simulink model "AtoD_test_FBand"  (R2016b)
settings: Solver=ode45  StartTime=0.0  StopTime=10.0  RelTol=1e-3
values from neighbouring files (symbols this model uses):
  Ts = 1/Fadc    (= 3.25520833333e-09)    [setupCryoFPGA.m]    (also in setupCryoFPGA_CMB.m; setupCryoFPGAorig.m = 3.2e-09)
undefined symbols (not defined in the file or in its folder): AXI4, Lite
libraries: xbsIndex_r4 x78
settings Model: Creator=ssmith  LastModifiedBy=jedu
settings DataIOCC: LimitDataPoints=on  SaveFormat=Array
settings OptimizationCC: BlockReduction=off  BooleanDataType=off  LifeSpan=inf
settings DebuggingCC: SaveWithParameterizedLinksMsg=none  UnderspecifiedInitializationDetection=Classic  MergeDetectMultiDrivingBlocksExec=none  SignalResolutionControl=TryResolveAllWithWarning  SFUnexpectedBacktrackingDiag=warning  SFNoUnconditionalDefaultTransitionDiag=warning  SFExecutionAtInitializationDiag=none
settings HardwareCC: ProdBitPerPointer=32  ProdBitPerSizeT=32  ProdBitPerPtrDiffT=32  ProdLargestAtomicFloat=None  ProdIntDivRoundTo=Undefined  ProdEndianess=Unspecified  ProdWordSize=32  ProdHWDeviceType=32-bit Generic  TargetUnknown=on
settings ModelReferenceCC: PropagateSignalLabelsOutOfModel=off
settings GRTTargetCC: TargetLangStandard=C89/C90 (ANSI)  GeneratePreprocessorConditionals=Disable all
settings ConfigComp: CovMetricSettings=dw  CovHtmlReporting=on  CovSaveCumulativeToWorkspaceVar=on  CovSaveSingleToWorkspaceVar=on  CovExternalEMLEnable=off  CovSFcnEnable=off

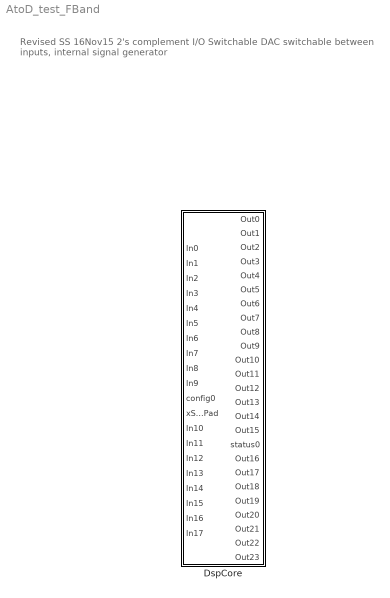
== system AtoD_test_FBand ==
  note: Revised SS 16Nov15
      | 	2's complement I/O
      | 	Switchable DAC switchable between inputs, internal signal generator
  DspCore : Subsystem

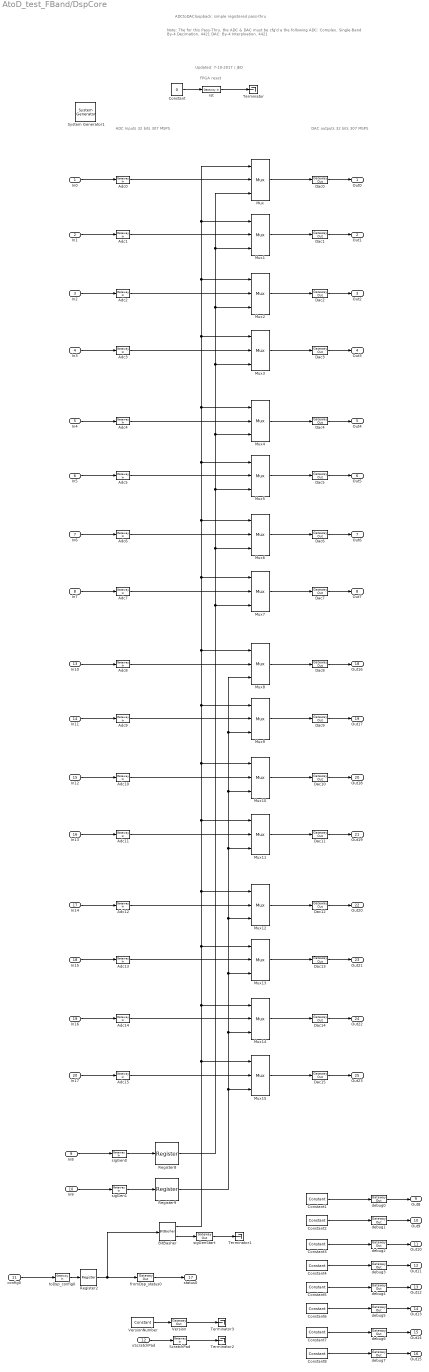
== system AtoD_test_FBand/DspCore ==
  note: Updated: 7-10-2017 / JED
  note: ADCtoDACloopback: simple registered pass-thru
  note: DAC outputs
      | 32 bits
      | 307 MSPS
  note: ADC Inputs
      | 32 bits
      | 307 MSPS
  note: FPGA reset
  note: Note: The for this Pass-Thru, the ADC & DAC must be cfg'd a the following
      |
      | ADC: Complex, Single-Band By-4 Decimation, 4421
      | DAC: By-4 Interploation, 4421
  In0 : Inport
  In1 : Inport  Port=2
  In2 : Inport  Port=3
  In3 : Inport  Port=4
  In4 : Inport  Port=5
  In5 : Inport  Port=6
  In6 : Inport  Port=7
  In7 : Inport  Port=8
  In8 : Inport  Port=9
  In9 : Inport  Port=10
  config0 : Inport  Port=11
  xScratchPad : Inport  Port=12
  In10 : Inport  Port=13
  In11 : Inport  Port=14
  In12 : Inport  Port=15
  In13 : Inport  Port=16
  In14 : Inport  Port=17
  In15 : Inport  Port=18
  In16 : Inport  Port=19
  In17 : Inport  Port=20
  " System Generator1" : xbsIndex_r4/ System Generator  Tag=genX  xilinxfamily=kintexu  part=xcku060  speed=-2-e  package=ffva1156  synthesis_tool=Vivado  clock_wrapper=Clock Enables  directory=./netlist  proj_type=Vivado  Synth_file=Vivado Synthesis Defaults  Impl_file=Vivado Implementation Defaults  testbench=off  simulink_period=Ts  sysclk_period=Ts*1e9  dcm_input_clock_period=10  incr_netlist=off  trim_vbits=Everywhere in SubSystem  dbl_ovrd=According to Block Masks  core_generation=According to Block Masks  run_coregen=off  deprecated_control=off  eval_field=0  block_type=sysgen
  Adc{0..15} (16 alike) : xbsIndex_r4/Gateway In  gui_display_data_type=Fixed-point  arith_type=Unsigned  n_bits=32  bin_pt=0  preci_type=Single  exp_width=8  frac_width=24  rows=1  columns=1  quantization=Truncate  overflow=Wrap  period=Ts  UseAsADC=off  ADCChannel='1'  interface=None  automatic_assignment=on  address_offset=hex2dec('00')  intf_name=''  intf_description=''  default_value=0  timing_constraint=None  locs_specified=off  LOCs={}  io_standard={}  inherit_from_input=off  hdl_port=on  dbl_ovrd=off  block_type=gatewayin
  BitBasher : xbsIndex_r4/BitBasher  bitexpr=|  display_expr=off  sr_1=sel  arith_type1=Unsigned  bin_pt1=0  sr_2=start  arith_type2=Unsigned  bin_pt2=0  sr_3=3  arith_type3=Unsigned  bin_pt3=0  sr_4=4  arith_type4=Unsigned  bin_pt4=0  dbl_ovrd=off  block_type=bitbasher
      | sel={a[0]}
      | start={a[1]}
  Constant : Constant  Value=0
  Constant1 : xbsIndex_r4/Constant  const=0  gui_display_data_type=Fixed-point  arith_type=Unsigned  n_bits=32  bin_pt=0  preci_type=Single  exp_width=8  frac_width=24  explicit_period=off  period=1  equ=P=C  opselect=C  inp2=PCIN>>17  opr=+  inp1=P  carry=CIN  dbl_ovrd=off  block_type=constant
  Constant2 : xbsIndex_r4/Constant  const=1  gui_display_data_type=Fixed-point  arith_type=Unsigned  n_bits=32  bin_pt=0  preci_type=Single  exp_width=8  frac_width=24  explicit_period=off  period=1  equ=P=C  opselect=C  inp2=PCIN>>17  opr=+  inp1=P  carry=CIN  dbl_ovrd=off  block_type=constant
  Constant3 : xbsIndex_r4/Constant  const=2  gui_display_data_type=Fixed-point  arith_type=Unsigned  n_bits=32  bin_pt=0  preci_type=Single  exp_width=8  frac_width=24  explicit_period=off  period=1  equ=P=C  opselect=C  inp2=PCIN>>17  opr=+  inp1=P  carry=CIN  dbl_ovrd=off  block_type=constant
  Constant4 : xbsIndex_r4/Constant  const=3  gui_display_data_type=Fixed-point  arith_type=Unsigned  n_bits=32  bin_pt=0  preci_type=Single  exp_width=8  frac_width=24  explicit_period=off  period=1  equ=P=C  opselect=C  inp2=PCIN>>17  opr=+  inp1=P  carry=CIN  dbl_ovrd=off  block_type=constant
  Constant5 : xbsIndex_r4/Constant  const=4  gui_display_data_type=Fixed-point  arith_type=Unsigned  n_bits=32  bin_pt=0  preci_type=Single  exp_width=8  frac_width=24  explicit_period=off  period=1  equ=P=C  opselect=C  inp2=PCIN>>17  opr=+  inp1=P  carry=CIN  dbl_ovrd=off  block_type=constant
  Constant6 : xbsIndex_r4/Constant  const=5  gui_display_data_type=Fixed-point  arith_type=Unsigned  n_bits=32  bin_pt=0  preci_type=Single  exp_width=8  frac_width=24  explicit_period=off  period=1  equ=P=C  opselect=C  inp2=PCIN>>17  opr=+  inp1=P  carry=CIN  dbl_ovrd=off  block_type=constant
  Constant7 : xbsIndex_r4/Constant  const=6  gui_display_data_type=Fixed-point  arith_type=Unsigned  n_bits=32  bin_pt=0  preci_type=Single  exp_width=8  frac_width=24  explicit_period=off  period=1  equ=P=C  opselect=C  inp2=PCIN>>17  opr=+  inp1=P  carry=CIN  dbl_ovrd=off  block_type=constant
  Constant8 : xbsIndex_r4/Constant  const=7  gui_display_data_type=Fixed-point  arith_type=Unsigned  n_bits=32  bin_pt=0  preci_type=Single  exp_width=8  frac_width=24  explicit_period=off  period=1  equ=P=C  opselect=C  inp2=PCIN>>17  opr=+  inp1=P  carry=CIN  dbl_ovrd=off  block_type=constant
  Dac{0..15} (16 alike) : xbsIndex_r4/Gateway Out  inherit_from_input=on  hdl_port=on  rows=1  columns=1  UseAsDAC=off  DACChannel='1'  interface=None  automatic_assignment=on  address_offset=hex2dec('00')  intf_name=''  intf_description=''  timing_constraint=None  locs_specified=off  LOCs={}  io_standard={}  block_type=gatewayout
  Mux{,1..15} (16 alike) : xbsIndex_r4/Mux  inputs=2  en=off  latency=1  precision=Full  arith_type=Unsigned  n_bits=16  bin_pt=14  quantization=Truncate  overflow=Wrap  dbl_ovrd=off  block_type=mux
  Register2 : xbsIndex_r4/Register  init=0  rst=off  en=off  dbl_ovrd=off  block_type=register
  Register8 : xbsIndex_r4/Register  init=0  rst=off  en=off  dbl_ovrd=off  block_type=register
  Register9 : xbsIndex_r4/Register  init=0  rst=off  en=off  dbl_ovrd=off  block_type=register
  ScratchPad : xbsIndex_r4/Gateway In  gui_display_data_type=Fixed-point  arith_type=Unsigned  n_bits=32  bin_pt=0  preci_type=Single  exp_width=8  frac_width=24  rows=1  columns=1  quantization="Round  (unbiased: +/- Inf)"  overflow=Saturate  period=Ts  UseAsADC=off  ADCChannel='1'  interface=AXI4-Lite  automatic_assignment=off  address_offset=hex2dec('FFC')  intf_name=''  intf_description=''  default_value=0  timing_constraint=None  locs_specified=off  LOCs={}  io_standard={}  inherit_from_input=off  hdl_port=on  dbl_ovrd=off  block_type=gatewayin
  Terminator{,1..3} (4 alike) : Terminator
  Version : xbsIndex_r4/Gateway Out  inherit_from_input=on  hdl_port=on  rows=1  columns=1  UseAsDAC=off  DACChannel='1'  interface=AXI4-Lite  automatic_assignment=off  address_offset=hex2dec('000')  intf_name=''  intf_description=''  timing_constraint=None  locs_specified=off  LOCs={}  io_standard={}  block_type=gatewayout
  VersionNumber : xbsIndex_r4/Constant  const=hex2dec('00000001')  gui_display_data_type=Fixed-point  arith_type=Unsigned  n_bits=32  bin_pt=0  preci_type=Single  exp_width=8  frac_width=24  explicit_period=off  period=1  equ=P=C  opselect=C  inp2=PCIN>>17  opr=+  inp1=P  carry=CIN  dbl_ovrd=off  block_type=constant
  debug{0..7} (8 alike) : xbsIndex_r4/Gateway Out  inherit_from_input=on  hdl_port=on  rows=1  columns=1  UseAsDAC=off  DACChannel='1'  interface=None  automatic_assignment=on  address_offset=hex2dec('00')  intf_name=''  intf_description=''  timing_constraint=None  locs_specified=off  LOCs={}  io_standard={}  block_type=gatewayout
  fromDsp_status0 : xbsIndex_r4/Gateway Out  inherit_from_input=on  hdl_port=on  rows=1  columns=1  UseAsDAC=off  DACChannel='1'  interface=AXI4-Lite  automatic_assignment=off  address_offset=hex2dec('004')  intf_name=''  intf_description=''  timing_constraint=None  locs_specified=off  LOCs={}  io_standard={}  block_type=gatewayout
  rst : xbsIndex_r4/Gateway In  gui_display_data_type=Boolean  arith_type=Boolean  n_bits=16  bin_pt=14  preci_type=Single  exp_width=8  frac_width=24  rows=1  columns=1  quantization="Round  (unbiased: +/- Inf)"  overflow=Saturate  period=Ts  UseAsADC=off  ADCChannel='1'  interface=None  automatic_assignment=on  address_offset=hex2dec('00')  intf_name=''  intf_description=''  default_value=0  timing_constraint=None  locs_specified=off  LOCs={}  io_standard={}  inherit_from_input=off  hdl_port=on  dbl_ovrd=off  block_type=gatewayin
  sigGen0 : xbsIndex_r4/Gateway In  gui_display_data_type=Fixed-point  arith_type=Unsigned  n_bits=32  bin_pt=0  preci_type=Single  exp_width=8  frac_width=24  rows=1  columns=1  quantization=Truncate  overflow=Wrap  period=Ts  UseAsADC=off  ADCChannel='1'  interface=None  automatic_assignment=on  address_offset=hex2dec('00')  intf_name=''  intf_description=''  default_value=0  timing_constraint=None  locs_specified=off  LOCs={}  io_standard={}  inherit_from_input=off  hdl_port=on  dbl_ovrd=off  block_type=gatewayin
  sigGen1 : xbsIndex_r4/Gateway In  gui_display_data_type=Fixed-point  arith_type=Unsigned  n_bits=32  bin_pt=0  preci_type=Single  exp_width=8  frac_width=24  rows=1  columns=1  quantization=Truncate  overflow=Wrap  period=Ts  UseAsADC=off  ADCChannel='1'  interface=None  automatic_assignment=on  address_offset=hex2dec('00')  intf_name=''  intf_description=''  default_value=0  timing_constraint=None  locs_specified=off  LOCs={}  io_standard={}  inherit_from_input=off  hdl_port=on  dbl_ovrd=off  block_type=gatewayin
  sigGenStart : xbsIndex_r4/Gateway Out  inherit_from_input=on  hdl_port=on  rows=1  columns=1  UseAsDAC=off  DACChannel='1'  interface=None  automatic_assignment=off  address_offset=hex2dec('004')  intf_name=''  intf_description=''  timing_constraint=None  locs_specified=off  LOCs={}  io_standard={}  block_type=gatewayout
  toDsp_config0 : xbsIndex_r4/Gateway In  gui_display_data_type=Fixed-point  arith_type=Unsigned  n_bits=32  bin_pt=0  preci_type=Single  exp_width=8  frac_width=24  rows=1  columns=1  quantization="Round  (unbiased: +/- Inf)"  overflow=Saturate  period=Ts  UseAsADC=off  ADCChannel='1'  interface=AXI4-Lite  automatic_assignment=off  address_offset=hex2dec('080')  intf_name=''  intf_description=''  default_value=0  timing_constraint=None  locs_specified=off  LOCs={}  io_standard={}  inherit_from_input=off  hdl_port=on  dbl_ovrd=off  block_type=gatewayin
  Out0 : Outport  OutDataTypeStr=uint32
  Out1 : Outport  Port=2
  Out2 : Outport  Port=3
  Out3 : Outport  Port=4
  Out4 : Outport  Port=5
  Out5 : Outport  Port=6
  Out6 : Outport  Port=7
  Out7 : Outport  Port=8
  Out8 : Outport  Port=9  OutDataTypeStr=uint32
  Out9 : Outport  Port=10  OutDataTypeStr=uint32
  Out10 : Outport  Port=11  OutDataTypeStr=uint32
  Out11 : Outport  Port=12  OutDataTypeStr=uint32
  Out12 : Outport  Port=13  OutDataTypeStr=uint32
  Out13 : Outport  Port=14  OutDataTypeStr=uint32
  Out14 : Outport  Port=15  OutDataTypeStr=uint32
  Out15 : Outport  Port=16  OutDataTypeStr=uint32
  status0 : Outport  Port=17
  Out16 : Outport  Port=18  OutDataTypeStr=uint32
  Out17 : Outport  Port=19
  Out18 : Outport  Port=20
  Out19 : Outport  Port=21
  Out20 : Outport  Port=22
  Out21 : Outport  Port=23
  Out22 : Outport  Port=24
  Out23 : Outport  Port=25
  wires:
  In0/1 -> Adc0/1
  Dac0/1 -> Out0/1
  Constant/1 -> rst/1
  rst/1 -> Terminator/1
  Adc0/1 -> Mux/2
  In1/1 -> Adc1/1
  Dac1/1 -> Out1/1
  Adc1/1 -> Mux1/2
  In2/1 -> Adc2/1
  Dac2/1 -> Out2/1
  Adc2/1 -> Mux2/2
  In3/1 -> Adc3/1
  Dac3/1 -> Out3/1
  Adc3/1 -> Mux3/2
  In4/1 -> Adc4/1
  Dac4/1 -> Out4/1
  Adc4/1 -> Mux4/2
  In5/1 -> Adc5/1
  Dac5/1 -> Out5/1
  Adc5/1 -> Mux5/2
  In6/1 -> Adc6/1
  Dac6/1 -> Out6/1
  Adc6/1 -> Mux6/2
  In7/1 -> Adc7/1
  Dac7/1 -> Out7/1
  Adc7/1 -> Mux7/2
  In8/1 -> sigGen0/1
  sigGen0/1 -> Register8/1
  In9/1 -> sigGen1/1
  sigGen1/1 -> Register9/1
  debug0/1 -> Out8/1
  debug1/1 -> Out9/1
  debug2/1 -> Out10/1
  debug3/1 -> Out11/1
  debug4/1 -> Out12/1
  debug5/1 -> Out13/1
  debug6/1 -> Out14/1
  debug7/1 -> Out15/1
  Constant1/1 -> debug0/1
  Constant2/1 -> debug1/1
  Constant3/1 -> debug2/1
  Constant4/1 -> debug3/1
  Constant5/1 -> debug4/1
  Constant6/1 -> debug5/1
  Constant7/1 -> debug6/1
  Constant8/1 -> debug7/1
  Mux/1 -> Dac0/1
  Mux1/1 -> Dac1/1
  Mux2/1 -> Dac2/1
  Mux3/1 -> Dac3/1
  Mux4/1 -> Dac4/1
  Mux5/1 -> Dac5/1
  Mux6/1 -> Dac6/1
  Mux7/1 -> Dac7/1
  Register9/1 -> Mux15/3, Mux14/3, Mux13/3, Mux12/3, Mux11/3, Mux10/3, Mux9/3, Mux8/3
  config0/1 -> toDsp_config0/1
  toDsp_config0/1 -> Register2/1
  fromDsp_status0/1 -> status0/1
  Register2/1 -> BitBasher/1, fromDsp_status0/1
  BitBasher/1 -> Mux15/1, Mux14/1, Mux13/1, Mux12/1, Mux11/1, Mux10/1, Mux9/1, Mux8/1, Mux7/1, Mux6/1, Mux5/1, Mux4/1, Mux3/1, Mux2/1, Mux1/1, Mux/1
  xScratchPad/1 -> ScratchPad/1
  ScratchPad/1 -> Terminator2/1
  Version/1 -> Terminator3/1
  VersionNumber/1 -> Version/1
  In10/1 -> Adc8/1
  Dac8/1 -> Out16/1
  Adc8/1 -> Mux8/2
  In11/1 -> Adc9/1
  Dac9/1 -> Out17/1
  Adc9/1 -> Mux9/2
  In12/1 -> Adc10/1
  Dac10/1 -> Out18/1
  Adc10/1 -> Mux10/2
  In13/1 -> Adc11/1
  Dac11/1 -> Out19/1
  Adc11/1 -> Mux11/2
  In14/1 -> Adc12/1
  Dac12/1 -> Out20/1
  Adc12/1 -> Mux12/2
  In15/1 -> Adc13/1
  Dac13/1 -> Out21/1
  Adc13/1 -> Mux13/2
  In16/1 -> Adc14/1
  Dac14/1 -> Out22/1
  Adc14/1 -> Mux14/2
  In17/1 -> Adc15/1
  Dac15/1 -> Out23/1
  Adc15/1 -> Mux15/2
  Mux8/1 -> Dac8/1
  Mux9/1 -> Dac9/1
  Mux10/1 -> Dac10/1
  Mux11/1 -> Dac11/1
  Mux12/1 -> Dac12/1
  Mux13/1 -> Dac13/1
  Mux14/1 -> Dac14/1
  Mux15/1 -> Dac15/1
  BitBasher/2 -> sigGenStart/1
  sigGenStart/1 -> Terminator1/1
  Register8/1 -> Mux7/3, Mux6/3, Mux5/3, Mux4/3, Mux3/3, Mux2/3, Mux1/3, Mux/3
